simulink model "problem1"  (R2020a)
settings: Solver=FixedStepDiscrete  StartTime=0.0  StopTime=200  RelTol=1e-3
settings Model: Creator=Riyansh  LastModifiedBy=Riyansh

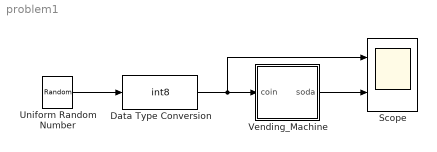
== system problem1 ==
  Data Type Conversion : DataTypeConversion  OutDataTypeStr=int8  RndMeth=Nearest  SaturateOnIntegerOverflow=on
  Scope : Scope  NumInputPorts=2
  Uniform Random Number : UniformRandomNumber  Minimum=0  Maximum=2  Seed=337  SampleTime=10
  Vending_Machine : Stateflow chart  TreatAsAtomicUnit=on
  wires:
  Data Type Conversion/1 -> Vending_Machine/1(coin), Scope/1
  Uniform Random Number/1 -> Data Type Conversion/1
  Vending_Machine/1(soda) -> Scope/2

== stateflow chart problem1/Vending_Machine ==
  settings: stateMachineType=MEALY_MACHINE  initializeOutput=1
  state got_0
  state got_nickel
  state got_dime
  (default) -> got_0
  got_0 -> got_nickel [order 1] : [coin==1]{soda=0}
  got_nickel -> got_0 [order 2] : [coin==2]{soda=1}
  got_dime -> got_0 [order 1] : [coin==1]{soda=1}
  got_0 -> got_dime [order 2] : [coin==2]{soda=0}
  got_nickel -> got_dime [order 1] : [coin==1]{soda=0}
  got_dime -> got_nickel [order 2] : [coin==2]{soda=1}
  data: coin input int8; soda output boolean
